simulink model "F_11_e"  (R2018a)
settings: Solver=VariableStepAuto  StartTime=0.0  StopTime=40  RelTol=1e-3
InitFcn:
  | vtol_param
  | F_11
StartFcn:
  | vtol_param
  | F_11
undefined symbols (not defined in the file or in its folder): P, PlotVtol, vtol_h_ctrl, vtol_z_ctrl
ContinueFcn:
  | FT2frfl
settings Model: Creator=sadam  LastModifiedBy=sadam

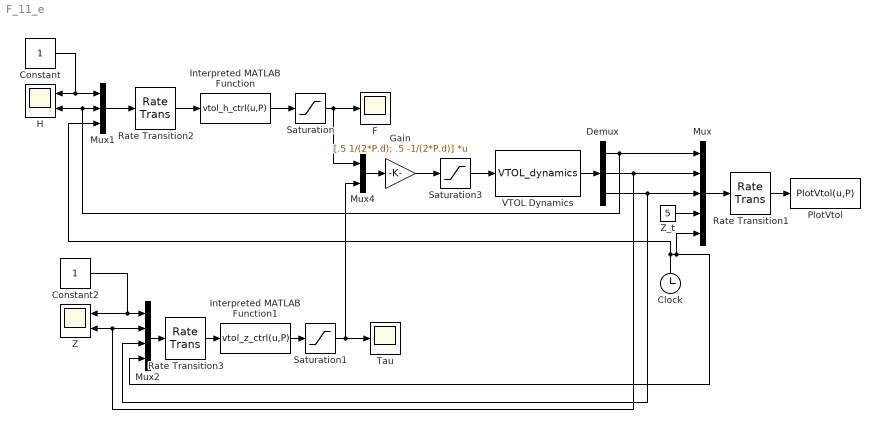
== system F_11_e ==
  Clock : Clock
  Constant : Constant
  Constant2 : Constant
  Demux : Demux  Outputs=3
  F : Scope
  Gain : Gain  Gain=[.5 1/(2*P.d); .5 -1/(2*P.d)]  Multiplication=Matrix(K*u)
  "H " : Scope  NumInputPorts=2
  Interpreted MATLAB Function : MATLABFcn  MATLABFcn=vtol_h_ctrl(u,P)
  Interpreted MATLAB Function1 : MATLABFcn  MATLABFcn=vtol_z_ctrl(u,P)
  Mux : Mux  Inputs=5
  Mux1 : Mux  Inputs=3
  Mux2 : Mux
  Mux4 : Mux  Inputs=2
  "PlotVtol " : MATLABFcn  MATLABFcn=PlotVtol(u,P)  OutputDimensions=0
  Rate Transition1 : RateTransition  OutPortSampleTime=P.t_plot
  Rate Transition2 : RateTransition  OutPortSampleTime=P.Ts
  Rate Transition3 : RateTransition  OutPortSampleTime=P.Ts
  Saturation : Saturate  UpperLimit=P.Force_max  LowerLimit=-P.Force_max
  Saturation1 : Saturate  UpperLimit=P.Torque_max  LowerLimit=-P.Torque_max
  Saturation3 : Saturate  UpperLimit=P.Force_max  LowerLimit=-P.Force_max
  Tau : Scope
  VTOL Dynamics : S-Function  FunctionName=VTOL_dynamics  Parameters=P  SFunctionDeploymentMode=off  EnableBusSupport=off
  Z : Scope  NumInputPorts=2
  Z_t : Constant  Value=5
  wires:
  Mux/1 -> Rate Transition1/1
  VTOL Dynamics/1 -> Demux/1
  Rate Transition1/1 -> "PlotVtol "/1
  Z_t/1 -> Mux/4
  Clock/1 -> Mux2/4, Mux/5, Mux1/3
  Demux/1 -> Mux/1, "H "/2, Mux1/2
  Demux/2 -> Mux/2, Z/2, Mux2/2
  Demux/3 -> Mux2/3, Mux/3
  Saturation3/1 -> VTOL Dynamics/1
  Gain/1 -> Saturation3/1
  Mux4/1 -> Gain/1
  Constant/1 -> "H "/1, Mux1/1
  Saturation/1 -> F/1, Mux4/1
  Interpreted MATLAB Function/1 -> Saturation/1
  Constant2/1 -> Z/1, Mux2/1
  Mux1/1 -> Rate Transition2/1
  Rate Transition2/1 -> Interpreted MATLAB Function/1
  Rate Transition3/1 -> Interpreted MATLAB Function1/1
  Interpreted MATLAB Function1/1 -> Saturation1/1
  Saturation1/1 -> Tau/1, Mux4/2
  Mux2/1 -> Rate Transition3/1
